simulink model "emo_a04_task"  (Simulink 7.5)
libraries: mathlib x16, reglib x4, speclib x1, genlib x1, arclib x1
settings Model: Creator=jsobota  LastModifiedBy=jsobota  ExtModeTrigMode=oneshot  ExtModeArmWhenConnect=off

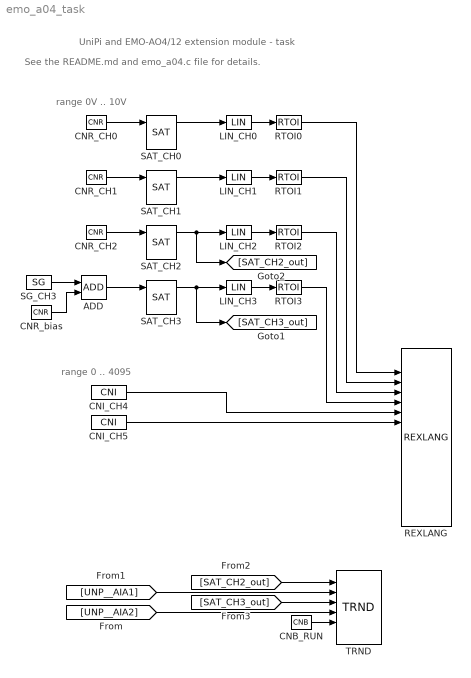
== system emo_a04_task ==
  note: range 0V .. 10V
  note: range 0 .. 4095
  note: See the README.md and emo_a04.c file for details.
  note: UniPi and EMO-AO4/12 extension module - task
  ADD : mathlib/ADD
  CNB_RUN : mathlib/CNB  YCN=on
  CNI_CH4 : mathlib/CNI  icn=1024
  CNI_CH5 : mathlib/CNI  icn=2048
  CNR_CH0 : mathlib/CNR  ycn=2.5
  CNR_CH1 : mathlib/CNR  ycn=5.0
  CNR_CH2 : mathlib/CNR  ycn=7.5
  CNR_bias : mathlib/CNR  ycn=5
  LIN_CH{0..3} (4 alike) : mathlib/LIN  u1=0  y1=0  u2=10  y2=4095
  REXLANG : speclib/REXLANG  strs=0  SystemSampleTime=-1  tab_matlab=BASIC  srcname=emo_a04.c  srctype=1: C-like  stack=0  debug=1: No check  p0=/dev/i2c-1  p1=0  p2=0  p3=0  p4=0  p5=0  p6=0  p7=0  p8=0  p9=0  p10=0  p11=0  p12=0  p13=0  p14=0  p15=0  fname=/dev/i2c-1
  RTOI{0..3} (4 alike) : mathlib/RTOI
  SAT_CH{0..3} (4 alike) : reglib/SAT  tp=0  tn=0  hilim0=10  lolim0=0  HLD=on
  SG_CH3 : genlib/SG  isig=1: SINE  amp=5  freq=0.1  phase=0  ifrunit=1: Hz  iphunit=1: degrees  offset=0
  TRND : arclib/TRND  n=4  l=1000  btype=8: Double  ptype1=1: Store  ptype2=1: Store  ptype3=1: Store  ptype4=1: Store  pfac=1  afac=0  arc=0  id=1  Title=Trend Title  timesrc=1
  wires:
  ADD/1 -> SAT_CH3/1
  CNB_RUN/1 -> TRND/5
  CNI_CH4/1 -> REXLANG/7
  CNI_CH5/1 -> REXLANG/8
  CNR_CH0/1 -> SAT_CH0/1
  CNR_CH1/1 -> SAT_CH1/1
  CNR_CH2/1 -> SAT_CH2/1
  CNR_bias/1 -> ADD/2
  [UNP__AIA2] -> TRND/4
  [UNP__AIA1] -> TRND/2
  [SAT_CH2_out] -> TRND/1
  [SAT_CH3_out] -> TRND/3
  LIN_CH0/1 -> RTOI0/1
  LIN_CH1/1 -> RTOI1/1
  LIN_CH2/1 -> RTOI2/1
  LIN_CH3/1 -> RTOI3/1
  RTOI0/1 -> REXLANG/3
  RTOI1/1 -> REXLANG/4
  RTOI2/1 -> REXLANG/5
  RTOI3/1 -> REXLANG/6
  SAT_CH0/1 -> LIN_CH0/1
  SAT_CH1/1 -> LIN_CH1/1
  SAT_CH2/1 -> [SAT_CH2_out], LIN_CH2/1
  SAT_CH3/1 -> [SAT_CH3_out], LIN_CH3/1
  SG_CH3/1 -> ADD/1
